simulink library "CLCDLookUp"  (R2020a)
settings: Solver=VariableStepAuto  StartTime=0.0  StopTime=10.0  RelTol=1e-3
undefined symbols (not defined in the file): aeroStruct
settings Model: Creator=John Jr  LastModifiedBy=John Jr

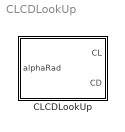
== system CLCDLookUp ==
  CLCDLookUp : Subsystem

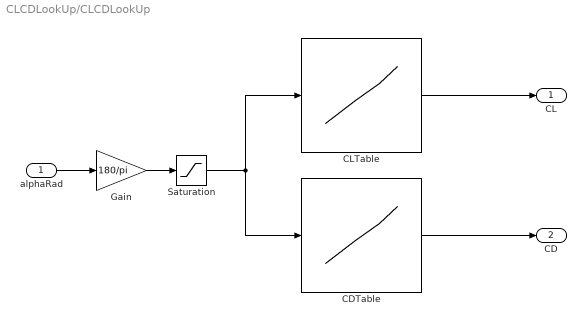
== system CLCDLookUp/CLCDLookUp ==
  alphaRad : Inport
  CDTable : Lookup_n-D  NumberOfTableDimensions=1  LookupTableObject=CLTable  BreakpointsForDimension1=aeroStruct.alpha  Table=aeroStruct.CD  ExtrapMethod=Clip  UseLastTableValue=on  InternalRulePriority=Speed  RndMeth=Simplest  InputSameDT=on
  CLTable : Lookup_n-D  NumberOfTableDimensions=1  LookupTableObject=CLTable  BreakpointsForDimension1=aeroStruct.alpha  Table=aeroStruct.CL  ExtrapMethod=Clip  UseLastTableValue=on  InternalRulePriority=Speed  RndMeth=Simplest  InputSameDT=on
  Gain : Gain  Gain=180/pi
  Saturation : Saturate  UpperLimit=90  LowerLimit=-90
  CL : Outport
  CD : Outport  Port=2
  wires:
  Gain/1 -> Saturation/1
  Saturation/1 -> CLTable/1, CDTable/1
  CDTable/1 -> CD/1
  alphaRad/1 -> Gain/1
  CLTable/1 -> CL/1
